simulink model "sampleModel291smplify"  (R2021b)
settings: Solver=VariableStepAuto  StartTime=0.0  StopTime=10.0  RelTol=1e-3
libraries: simulink x1
settings Model: Creator=user  LastModifiedBy=cemery

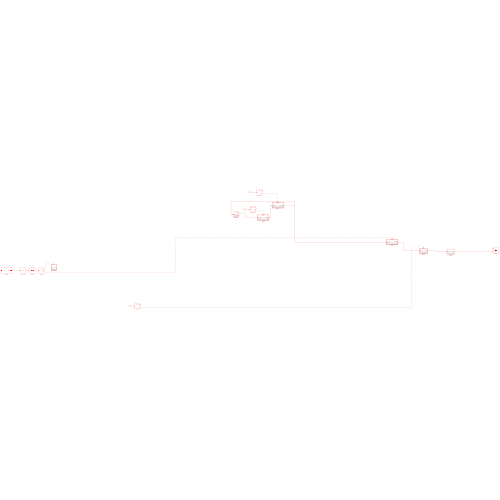
[thumbnail: Simulink's stored preview of the top-level diagram]
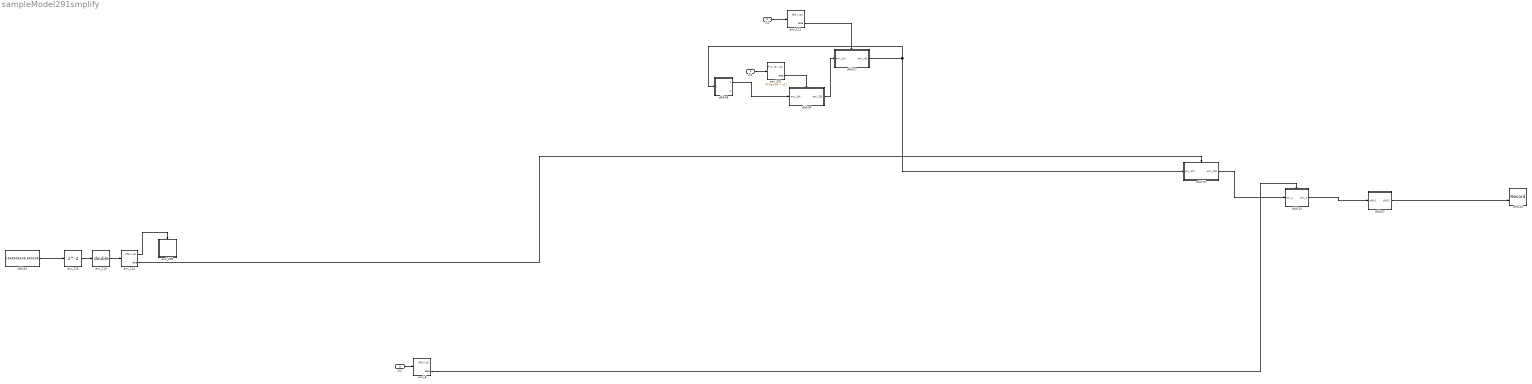
== system sampleModel291smplify ==
  In1 : Inport
  In2 : Inport  Port=2
  In3 : Inport  Port=3
  cfblk10 : Subsystem  TreatAsAtomicUnit=on
  cfblk27 : Subsystem  TreatAsAtomicUnit=on
  cfblk44 : Record  FileSettingsInternal="{\"entries\":[{\"content\":{\"excelSettings\":{\"content\":{},\"type\":\"Streamout.ExcelSettings\"}},\"type\":\"Streamout.FileSettingStorage\",\"uuid\":\"304e5b07-cea9-4883-a8e5-ec6bcf0d3d06\"}],\"packageUris\":[\"http://schema.mathworks.com/mf0/streamout_blocks/R2020a\"],\"version\":\"1.0\"}"  Layout=[1 1]  SignalsInternal="{\"entries\":[{\"content\":{\"signals\":[{\"content\":{\"blockPath\":[\"sampleModel291_pp_618_1_difftest/cfblk44\"],\"channel\":[],\"dimensions\":[1],\"domain\":\"sampleModel291_pp_618_1_difftest/cfblk44\",\"lineColor\":\"#fe330a\",\"plots\":[],\"port\":2,\"sid\":[\"\"],\"signalID\":99089,\"signalName\":\"cfblk67\"},\"type\":\"RecordBlkView.Signal\",\"uuid\":\"e41c9464-13b2-4b25-8d39-bb65eb09fde0\"},{\"content\":{\"blockPath\":[\"sampleModel291_pp_618_1_difftest/cfblk44\"],\"channel\":[],\"dimensions\":[1],\"domain\":\"sampleModel291_pp_618_1_difftest/cfblk44\",\"lineColor\":\"#0072bd\",\"plots\":[],\"port\":1,\"sid\":[\"\"],\"signalID\":99093},\"type\":\"RecordBlkView.Signal\",\"uuid\":\"b770d662-9053-4867-a5d0-5fbeb7da3783\"}]},\"type\":\"RecordBlkView.InputSignals\",\"uuid\":\"48eb4e34-f8ec-4e84-9ec4-8688e1f67d7c\"}],\"packageUris\":[\"http://schema.mathworks.com/mf0/streamout_blocks/R2020a\"],\"version\":\"1.0\"}"  VisualizationBindings="{\"xyplotplugin\":{\"info\":[{\"series\":[],\"subplotID\":1}]}}"  CompatibilityTag=XY
  cfblk54 : Constant  Value=[548506146.640336]  SampleTime=1
  cfblk67 : Subsystem
  cfblk68 : Subsystem
  cfblk75 : Subsystem  TreatAsAtomicUnit=on
  cfblk94 : Subsystem  TreatAsAtomicUnit=on
  emi_111 : If  IfExpression=0 > u1
  emi_209 : Subsystem  TreatAsAtomicUnit=on
  emi_214 : If  IfExpression=0 > u1  SampleTime=[1 0]
  emi_215 : DataTypeConversion  OutDataTypeStr=double
  emi_216 : Delay  InitialCondition=548506146.6403  SampleTime=1
  emi_291 : If  IfExpression=-1e+09 > u1  SampleTime=[1 0]
  emi_8 : If  IfExpression=0 > u1  SampleTime=[1 0]
  wires:
  cfblk68/1(cfblk2) -> cfblk94/1(emi_284)
  emi_291/2 -> cfblk94/Action
  cfblk10/1(emi_2) -> cfblk67/1(cfblk1)
  emi_214/1 -> emi_209/Action
  emi_216/1 -> emi_215/1
  emi_215/1 -> emi_214/1
  emi_214/2 -> cfblk75/Action
  cfblk75/1(emi_208) -> cfblk10/1(emi_1)
  emi_111/2 -> cfblk27/Action
  emi_8/2 -> cfblk10/Action
  cfblk67/1(cfblk2) -> cfblk44/2
  cfblk27/1(emi_105) -> cfblk68/1(cfblk1), cfblk75/1(emi_207)
  cfblk94/1(emi_285) -> cfblk27/1(emi_104)
  cfblk54/1 -> emi_216/1
  In1/1 -> emi_291/1
  In2/1 -> emi_111/1
  In3/1 -> emi_8/1

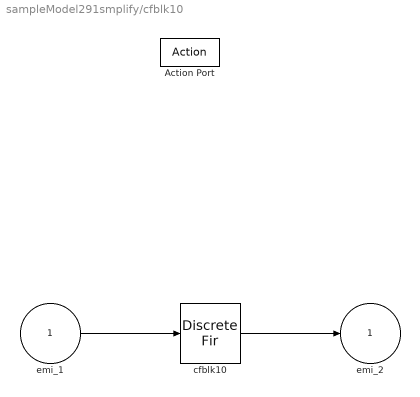
== system sampleModel291smplify/cfblk10 ==
  emi_1 : Inport
  Action Port : ActionPort  ActionPortLabel=else
  cfblk10 : DiscreteFir  SampleTime=1
  emi_2 : Outport
  wires:
  emi_1/1 -> cfblk10/1
  cfblk10/1 -> emi_2/1

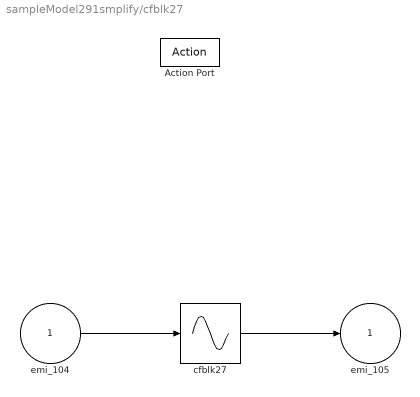
== system sampleModel291smplify/cfblk27 ==
  emi_104 : Inport
  Action Port : ActionPort  ActionPortLabel=else
  cfblk27 : Sin  TimeSource=Use external signal  SampleTime=0
  emi_105 : Outport
  wires:
  emi_104/1 -> cfblk27/1
  cfblk27/1 -> emi_105/1

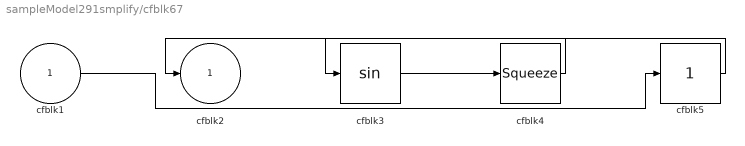
== system sampleModel291smplify/cfblk67 ==
  cfblk1 : Inport
  cfblk3 : Trigonometry
  cfblk4 : Squeeze
  cfblk5 : simulink/Math Operations/Slider Gain  gain=1  low=0  high=2
  cfblk2 : Outport
  wires:
  cfblk4/1 -> cfblk2/1
  cfblk1/1 -> cfblk5/1
  cfblk3/1 -> cfblk4/1
  cfblk5/1 -> cfblk3/1

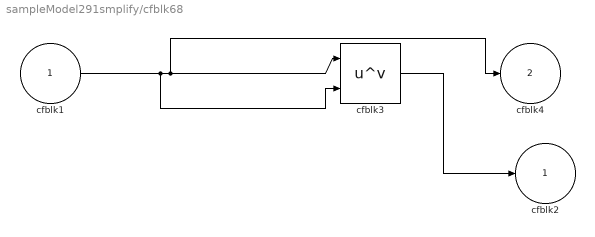
== system sampleModel291smplify/cfblk68 ==
  cfblk1 : Inport
  cfblk3 : Math  Operator=pow  SaturateOnIntegerOverflow=on
  cfblk2 : Outport
  cfblk4 : Outport  Port=2
  wires:
  cfblk1/1 -> cfblk4/1, cfblk3/1, cfblk3/2
  cfblk3/1 -> cfblk2/1

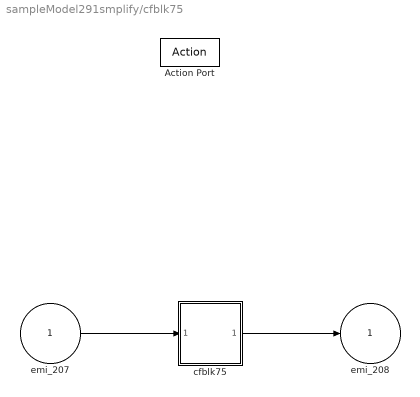
== system sampleModel291smplify/cfblk75 ==
  emi_207 : Inport
  Action Port : ActionPort  ActionPortLabel=else
  cfblk75 : Subsystem
  emi_208 : Outport
  wires:
  emi_207/1 -> cfblk75/1(cfblk1)
  cfblk75/1(cfblk2) -> emi_208/1

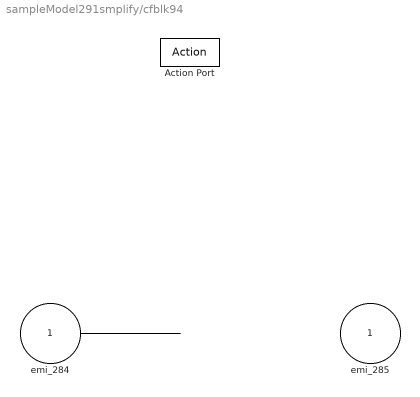
== system sampleModel291smplify/cfblk94 ==
  emi_284 : Inport
  Action Port : ActionPort  ActionPortLabel=else
  emi_285 : Outport
  wires:
  emi_284/1 -> ?
  ? -> emi_285/1

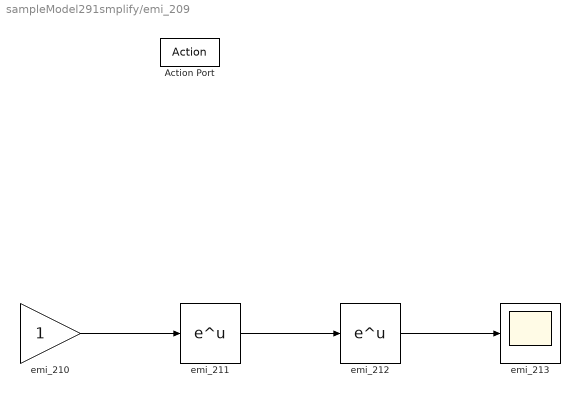
== system sampleModel291smplify/emi_209 ==
  Action Port : ActionPort  ActionPortLabel=if(0 > u1)
  emi_210 : Gain  SampleTime=[1 0]
  emi_211 : Math  SampleTime=[1 0]  SaturateOnIntegerOverflow=on
  emi_212 : Math  SampleTime=[1 0]  SaturateOnIntegerOverflow=on
  emi_213 : Scope
  wires:
  emi_210/1 -> emi_211/1
  emi_211/1 -> emi_212/1
  emi_212/1 -> emi_213/1

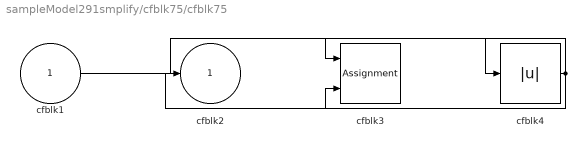
== system sampleModel291smplify/cfblk75/cfblk75 ==
  cfblk1 : Inport
  cfblk3 : Assignment  DiagnosticForDimensions=Warning  IndexOptions=Index vector (dialog)  Indices=1  OutputSizes=1
  cfblk4 : Abs
  cfblk2 : Outport
  wires:
  cfblk4/1 -> cfblk3/2, cfblk3/1, cfblk2/1
  cfblk1/1 -> cfblk4/1
